simulink subsystem "MagnetoField"  (R2021a)
settings: Solver=VariableStepAuto  StartTime=0.0  StopTime=10.0  RelTol=1e-3
undefined symbols (not defined in the file): WMM2020
libraries: aerolibgravity2 x1
settings Model: Creator=Laura  LastModifiedBy=Laura

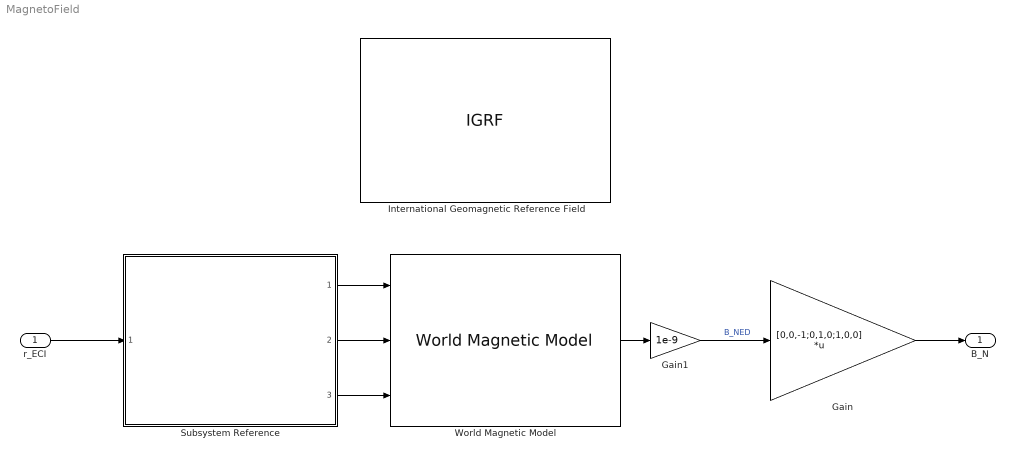
== system MagnetoField ==
  r_ECI : Inport
  Gain : Gain  Gain=[0,0,-1;0,1,0;1,0,0]  Multiplication=Matrix(K*u)
  Gain1 : Gain  Gain=1e-9
  International Geomagnetic Reference Field : IGRF  time_in=off  month=January  day=1  year=year  sv_out=off
      settings: AttributesFormatString=%<generation>
  Subsystem Reference : Subsystem  ReferencedSubsystem=ECI2GroundTrack
  World Magnetic Model : aerolibgravity2/World Magnetic Model  model=WMM2020 (2020-2025)  customFile='WMM2020.COF'  units=Metric (MKS)  time_in=off  month=January  day=1  year=year  action=Error  h_out=off  dec_out=off  inc_out=off  ti_out=off
      settings: SourceProductBaseCode=AE
  B_N : Outport
  wires:
  Subsystem Reference/3 -> World Magnetic Model/3
  Subsystem Reference/2 -> World Magnetic Model/2
  Subsystem Reference/1 -> World Magnetic Model/1
  r_ECI/1 -> Subsystem Reference/1
  World Magnetic Model/1 -> Gain1/1
  Gain1/1 -> Gain/1  "B_NED"
  Gain/1 -> B_N/1
